simulink model "expe1_model_v2"  (R2019b)
settings: Solver=VariableStepAuto  StartTime=0.0  StopTime=time  RelTol=1e-3
values from neighbouring files (symbols this model uses):
  D = Kc*tauD    (= 0.168)    [expe1_params_v2.m]
  Fds = tf([Kc*tauD 0], [beta*tauD 1])    [expe1_params_v2.m]
  Gs = tf(1, [1 3 3 1 0])    [expe1_params_v1.m]    (also in expe1_params_v2.m; expe2_params.m = tf([-1 0.4], [1 0.5 0.04]))
  half_time = time/2    (= 25)    [expe1_params_v1.m]    (also in expe1_params_v2.m = 250; expe2_params.m = 50)
  I = Kc/tauI    (= 0.07)    [expe1_params_v2.m]
  Kc = 0.56    [expe1_params_v1.m]    (also in expe1_params_v2.m)
  LPF = tf(1, [beta*tauD 1])    [expe1_params_v2.m]
  P = Kc    (= 0.56)    [expe1_params_v1.m]    (also in expe1_params_v2.m)
  tauD = 0.3    [expe1_params_v1.m]    (also in expe1_params_v2.m)
  tauI = 8    [expe1_params_v1.m]    (also in expe1_params_v2.m)
  time = 50    [expe1_params_v1.m]    (also in expe1_params_v2.m = 500; expe2_params.m = 100)
libraries: simulink x3
settings Model: Creator=adityaaaap  LastModifiedBy=adityaaaap

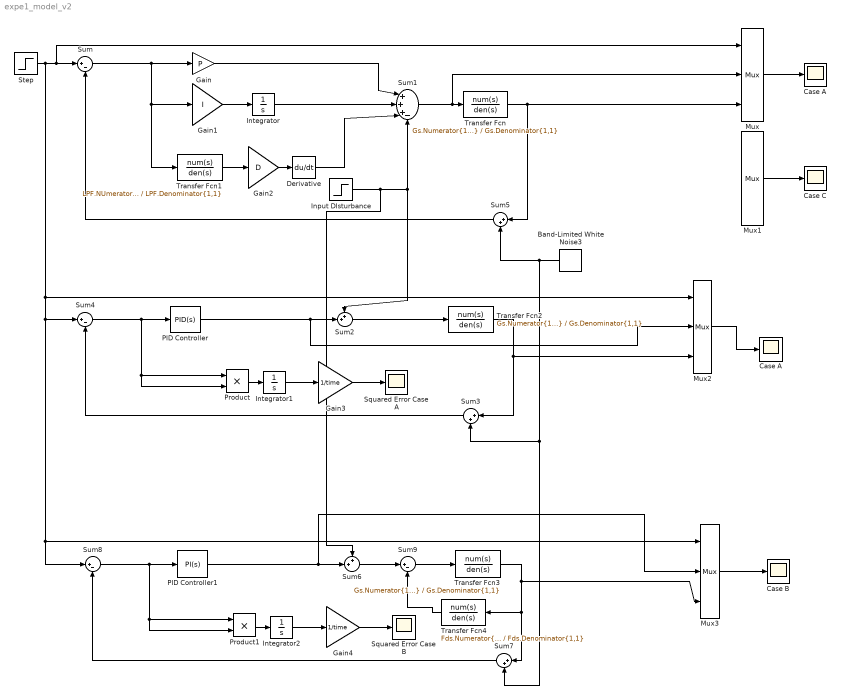
== system expe1_model_v2 ==
  Band-Limited White Noise3 : simulink/Sources/Band-Limited White Noise  Cov=[0.001]  Ts=0.1  seed=[23341]
  Case A : Scope
  "Case A " : Scope
  Case B : Scope
  Case C : Scope
  Derivative : Derivative
  Gain : Gain  Gain=P
  Gain1 : Gain  Gain=I
  Gain2 : Gain  Gain=D
  Gain3 : Gain  Gain=1/time
  Gain4 : Gain  Gain=1/time
  Input DIsturbance : Step  Time=half_time  After=-3  SampleTime=0
  Integrator : Integrator
  Integrator1 : Integrator
  Integrator2 : Integrator
  Mux{,1..3} (4 alike) : Mux  Inputs=3
  PID Controller : simulink/Continuous/PID Controller  Controller=PID  Form=Parallel  TimeDomain=Continuous-time  SampleTime=-1  IntegratorMethod=Forward Euler  FilterMethod=Forward Euler  ControllerParametersSource=internal  P=Kc  I=Kc/tauI  D=Kc*tauD  UseFilter=on  N=1/(0.1*tauD)  TunerSelectOption=Transfer Function Based (PID Tuner App)  InitialConditionSource=internal  InitialConditionForIntegrator=0  InitialConditionForFilter=0  DifferentiatorICPrevScaledInput=0  ExternalReset=none  TrackingMode=off  Kt=1  LimitOutput=off  UpperSaturationLimit=inf  LowerSaturationLimit=-inf  LinearizeAsGain=on  AntiWindupMode=none  Kb=1  POutMin=[]  POutMax=[]  IOutMin=[]  IOutMax=[]  DOutMin=[]  DOutMax=[]  NOutMin=[]  NOutMax=[]  SumOutMin=[]  SumOutMax=[]  SaturationOutMin=[]  SaturationOutMax=[]  PParamMin=[]  PParamMax=[]  IParamMin=[]  IParamMax=[]  DParamMin=[]  DParamMax=[]  NParamMin=[]  NParamMax=[]  KbParamMin=[]  KbParamMax=[]  KtParamMin=[]  KtParamMax=[]  KbOutMin=[]  KbOutMax=[]  KtOutMin=[]  KtOutMax=[]  IntegratorOutMin=[]  IntegratorOutMax=[]  FilterOutMin=[]  FilterOutMax=[]  SumI1OutMin=[]  SumI1OutMax=[]  SumI2OutMin=[]  SumI2OutMax=[]  SumI3OutMin=[]  SumI3OutMax=[]  SumI4OutMin=[]  SumI4OutMax=[]  SumDOutMin=[]  SumDOutMax=[]  DifferentiatorOutMin=[]  DifferentiatorOutMax=[]  FilterDiffOutCoefMin=[]  FilterDiffOutCoefMax=[]  ReciprocalOutMin=[]  ReciprocalOutMax=[]  SumDenOutMin=[]  SumDenOutMax=[]  SumNumOutMin=[]  SumNumOutMax=[]  DivideOutMin=[]  DivideOutMax=[]  IntegratorContinuousStateAttributes=''  IntegratorStateMustResolveToSignalObject=off  IntegratorRTWStateStorageClass=Auto  FilterContinuousStateAttributes=''  FilterStateMustResolveToSignalObject=off  FilterRTWStateStorageClass=Auto  ParallelPVariant=InternalParameters  IdealPVariant=Disabled  IVariant=InternalParameters  DVariant=InternalParameters  IntegratorVariant=Continuous  SatVariant=Disabled  AWVariant=Passthrough  PCopyVariant=Disabled  TRVariant=Disabled  FdbkBlocksVariant=Forward  IdealPFdbkVariant=Disabled  SatFdbkVariant=Disabled  DerivativeFilterVariant=ContFilter  NVariant=InternalParameters  NCopyVariant=Disabled  FilterICVariant=InternalICsFilter  IntegratorICVariant=InternalICs  ExternalResetVariant=Disabled  TRSumVariant=Passthrough  SumFdbkVariant=Disabled  SumVariant=Sum_PID
  PID Controller1 : simulink/Continuous/PID Controller  Controller=PI  Form=Parallel  TimeDomain=Continuous-time  SampleTime=-1  IntegratorMethod=Forward Euler  FilterMethod=Forward Euler  ControllerParametersSource=internal  P=Kc  I=Kc/tauI  D=Kc*tauD  UseFilter=on  N=1/(0.1*tauD)  TunerSelectOption=Transfer Function Based (PID Tuner App)  InitialConditionSource=internal  InitialConditionForIntegrator=0  InitialConditionForFilter=0  DifferentiatorICPrevScaledInput=0  ExternalReset=none  TrackingMode=off  Kt=1  LimitOutput=off  UpperSaturationLimit=inf  LowerSaturationLimit=-inf  LinearizeAsGain=on  AntiWindupMode=none  Kb=1  POutMin=[]  POutMax=[]  IOutMin=[]  IOutMax=[]  DOutMin=[]  DOutMax=[]  NOutMin=[]  NOutMax=[]  SumOutMin=[]  SumOutMax=[]  SaturationOutMin=[]  SaturationOutMax=[]  PParamMin=[]  PParamMax=[]  IParamMin=[]  IParamMax=[]  DParamMin=[]  DParamMax=[]  NParamMin=[]  NParamMax=[]  KbParamMin=[]  KbParamMax=[]  KtParamMin=[]  KtParamMax=[]  KbOutMin=[]  KbOutMax=[]  KtOutMin=[]  KtOutMax=[]  IntegratorOutMin=[]  IntegratorOutMax=[]  FilterOutMin=[]  FilterOutMax=[]  SumI1OutMin=[]  SumI1OutMax=[]  SumI2OutMin=[]  SumI2OutMax=[]  SumI3OutMin=[]  SumI3OutMax=[]  SumI4OutMin=[]  SumI4OutMax=[]  SumDOutMin=[]  SumDOutMax=[]  DifferentiatorOutMin=[]  DifferentiatorOutMax=[]  FilterDiffOutCoefMin=[]  FilterDiffOutCoefMax=[]  ReciprocalOutMin=[]  ReciprocalOutMax=[]  SumDenOutMin=[]  SumDenOutMax=[]  SumNumOutMin=[]  SumNumOutMax=[]  DivideOutMin=[]  DivideOutMax=[]  IntegratorContinuousStateAttributes=''  IntegratorStateMustResolveToSignalObject=off  IntegratorRTWStateStorageClass=Auto  FilterContinuousStateAttributes=''  FilterStateMustResolveToSignalObject=off  FilterRTWStateStorageClass=Auto  ParallelPVariant=InternalParameters  IdealPVariant=Disabled  IVariant=InternalParameters  DVariant=Disabled  IntegratorVariant=Continuous  SatVariant=Disabled  AWVariant=Passthrough  PCopyVariant=Disabled  TRVariant=Disabled  FdbkBlocksVariant=Forward  IdealPFdbkVariant=Disabled  SatFdbkVariant=Disabled  DerivativeFilterVariant=Disabled  NVariant=Disabled  NCopyVariant=Disabled_SignalSpec  FilterICVariant=Disabled  IntegratorICVariant=InternalICs  ExternalResetVariant=Disabled  TRSumVariant=Passthrough  SumFdbkVariant=Disabled  SumVariant=Sum_PI
  Product : Product
  Product1 : Product
  Squared Error Case A : Scope
  Squared Error Case B : Scope
  Step : Step  Time=0  After=6  SampleTime=0.1
  Sum{,4,8..9} (4 alike) : Sum  Inputs=|+-
  Sum1 : Sum  Inputs=|+++-
  Sum2 : Sum  Inputs=++|
  Sum3 : Sum  Inputs=|++
  Sum5 : Sum  Inputs=|++
  Sum6 : Sum  Inputs=++|
  Sum7 : Sum  Inputs=|++
  Transfer Fcn : TransferFcn  Numerator=Gs.Numerator{1,1}  Denominator=Gs.Denominator{1,1}
  Transfer Fcn1 : TransferFcn  Numerator=LPF.NUmerator{1,1}  Denominator=LPF.Denominator{1,1}
  Transfer Fcn2 : TransferFcn  Numerator=Gs.Numerator{1,1}  Denominator=Gs.Denominator{1,1}
  Transfer Fcn3 : TransferFcn  Numerator=Gs.Numerator{1,1}  Denominator=Gs.Denominator{1,1}
  Transfer Fcn4 : TransferFcn  Numerator=Fds.Numerator{1,1}  Denominator=Fds.Denominator{1,1}
  wires:
  Gain1/1 -> Integrator/1
  Gain2/1 -> Derivative/1
  Integrator/1 -> Sum1/2
  Mux/1 -> Case A/1
  Mux1/1 -> Case C/1
  Mux2/1 -> "Case A "/1
  Sum1/1 -> Mux/2, Transfer Fcn/1
  Transfer Fcn/1 -> Sum5/1, Mux/3
  Sum5/1 -> Sum/2
  Sum/1 -> Transfer Fcn1/1, Gain1/1, Gain/1
  Gain/1 -> Sum1/1
  Derivative/1 -> Sum1/3
  Transfer Fcn1/1 -> Gain2/1
  PID Controller/1 -> Sum2/2, Mux2/2
  Product/1 -> Integrator1/1
  Integrator1/1 -> Gain3/1
  Sum4/1 -> Product/2, Product/1, PID Controller/1
  Sum2/1 -> Transfer Fcn2/1
  Gain3/1 -> Squared Error Case A/1
  Transfer Fcn2/1 -> Sum3/1, Mux2/3
  Sum3/1 -> Sum4/2
  Mux3/1 -> Case B/1
  Sum8/1 -> Product1/2, Product1/1, PID Controller1/1
  Product1/1 -> Integrator2/1
  Integrator2/1 -> Gain4/1
  Step/1 -> Mux2/1, Sum8/1, Mux3/1, Sum4/1, Sum/1, Mux/1
  Input DIsturbance/1 -> Sum1/4, Sum2/1, Sum6/1
  PID Controller1/1 -> Sum6/2, Mux3/2
  Gain4/1 -> Squared Error Case B/1
  Sum6/1 -> Sum9/1
  Band-Limited White Noise3/1 -> Sum3/2, Sum7/2, Sum5/2
  Sum9/1 -> Transfer Fcn3/1
  Sum7/1 -> Sum8/2
  Transfer Fcn4/1 -> Sum9/2
  Transfer Fcn3/1 -> Transfer Fcn4/1, Sum7/1, Mux3/3
